simulink model "transmissionlineprotection1"  (R2017a)
settings: Solver=VariableStepAuto  StartTime=0.0  StopTime=0.25  RelTol=1e-3
libraries: powerlib x10, sdolib x6, simulink_extras x3, powerlib_meascontrol x1
settings Model: Creator=abhishek tiwari  LastModifiedBy=abhishek tiwari
settings DataIOCC: ReturnWorkspaceOutputs=on
settings DebuggingCC: UnconnectedInputMsg=none  UnconnectedOutputMsg=none  UnconnectedLineMsg=none
settings ModelReferenceCC: EnableRefExpFcnMdlSchedulingChecks=off
settings SFSimCC: SimUseLocalCustomCode=on
settings RTWCC: RTWUseLocalCustomCode=on

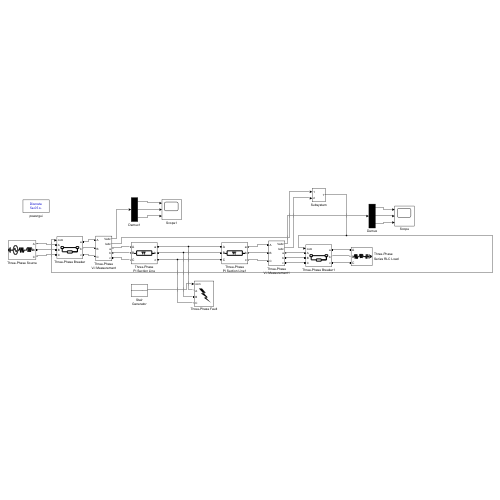
[thumbnail: Simulink's stored preview of the top-level diagram]
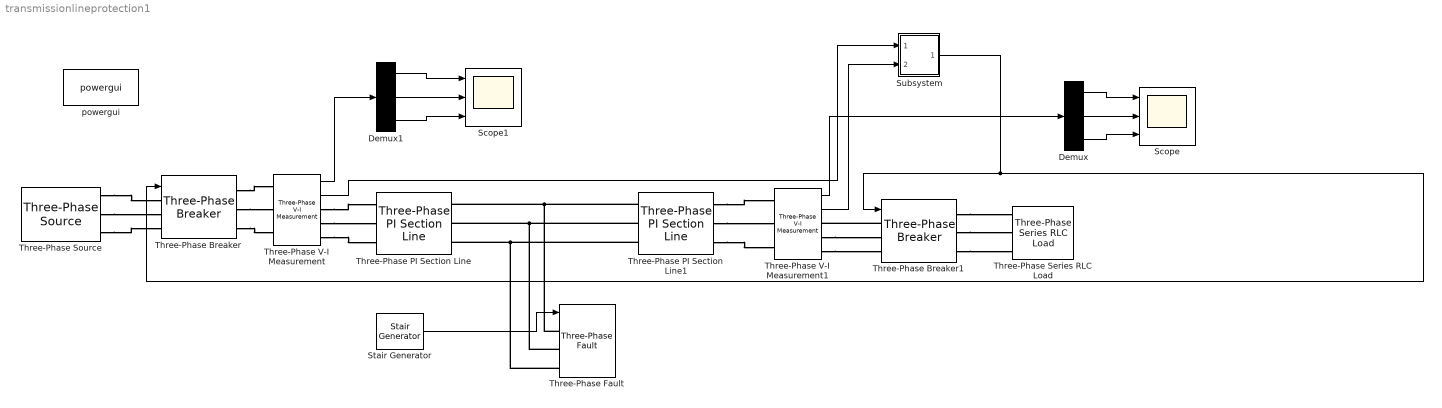
== system transmissionlineprotection1 ==
  Demux : Demux  Outputs=3
  Demux1 : Demux  Outputs=3
  Scope : Scope  NumInputPorts=3
  Scope1 : Scope  NumInputPorts=3
  Stair Generator : powerlib_meascontrol/Pulse & Signal Generators/Stair Generator  t=[0,0.02,0.14,0.2]  e=[0,0,0,0]  Ts=0
  Subsystem : Subsystem
  Three-Phase PI Section Line : powerlib/Elements/Three-Phase PI Section Line  LConnTagsString=a|b|c  RConnTagsString=A|B|C  Length=100  Frequency=50  Resistances=[ 0.01273 0.3864]  Inductances="[ 0.9337e-3  4.1264e-3]"  Capacitances=[12.74e-9 7.751e-9]
  Three-Phase PI Section Line1 : powerlib/Elements/Three-Phase PI Section Line  LConnTagsString=a|b|c  RConnTagsString=A|B|C  Length=100  Frequency=50  Resistances=[ 0.01273 0.3864]  Inductances="[ 0.9337e-3  4.1264e-3]"  Capacitances=[12.74e-9 7.751e-9]
  Three-Phase Series RLC Load : powerlib/Elements/Three-Phase Series RLC Load  LConnTagsString=A|B|C  Configuration=Y (grounded)  NominalVoltage=1000  Vabc=[1e3 1e3 1e3]  Vabcp=[1e3 1e3 1e3]  NominalFrequency=50  UnbalancedPower=off  ActivePower=10e3  InductivePower=100  CapacitivePower=100  Pabc=[10e3 9e3 11e3]  QLabc=[100 90 110]  QCabc=[100 90 110]  Pabcp=[10e3 9e3 11e3]  QLabcp=[100 90 110]  QCabcp=[100 90 110]  Measurements=None  LoadType=constant Z
  Three-Phase V-I Measurement : powerlib/Measurements/Three-Phase V-I Measurement  VoltageMeasurement=phase-to-ground  SetLabelV=off  LabelV=Vabc  Vpu=off  VpuLL=off  CurrentMeasurement=yes  SetLabelI=off  LabelI=Iabc  Ipu=off  Pbase=100e6  Vbase=500e3  OutputType=Complex  PhasorSimulation=off  PSBequivalent=0
  Three-Phase V-I Measurement1 : powerlib/Measurements/Three-Phase V-I Measurement  VoltageMeasurement=phase-to-ground  SetLabelV=off  LabelV=Vabc  Vpu=off  VpuLL=off  CurrentMeasurement=yes  SetLabelI=off  LabelI=Iabc  Ipu=off  Pbase=100e6  Vbase=500e3  OutputType=Complex  PhasorSimulation=off  PSBequivalent=0
  Three-Phase Breaker : powerlib/Elements/Three-Phase Breaker  InitialState=closed  SwitchA=on  SwitchB=on  SwitchC=on  SwitchTimes="[1/60  5/60]"  External=on  BreakerResistance=0.01  SnubberResistance=1e6  SnubberCapacitance=inf  Measurements=None
  Three-Phase Breaker1 : powerlib/Elements/Three-Phase Breaker  InitialState=closed  SwitchA=on  SwitchB=on  SwitchC=on  SwitchTimes="[1/60  5/60]"  External=on  BreakerResistance=0.01  SnubberResistance=1e6  SnubberCapacitance=inf  Measurements=None
  Three-Phase Fault : powerlib/Elements/Three-Phase Fault  InitialStates=0  FaultA=on  FaultB=on  FaultC=on  GroundFault=on  SwitchTimes="[1/60  5/60]"  External=on  SwitchStatus=NaN  FaultResistance=0.001  GroundResistance=0.01  SnubberResistance=1e6  SnubberCapacitance=inf  Measurements=None
  Three-Phase Source : powerlib/Electrical Sources/Three-Phase Source  InternalConnection=Yg  VoltagePhases=off  Voltage=25e3  PhaseAngle=0  Voltage_phases=[25e3 25e3 25e3]/sqrt(3)  PhaseAngles_phases=[0 -120 +120]  Frequency=50  NonIdealSource=on  SpecifyImpedance=on  Resistance=0.8929  Inductance=16.58e-3  ShortCircuitLevel=100e6  BaseVoltage=25e3  XRratio=7  BusType=swing  Pref=10e3  Qref=0  Prefabc=[10e3, 10e3, 10e3]  Qrefabc=[0, 0, 0]  Qmin=-inf  Qmax=inf
  powergui : powerlib/powergui  Priority=1  SimulationMode=Discrete  SampleTime=50e-6  frequency=60  Iterations=50  frequencyindice=50  Pbase=100e6  ErrMax=1e-4  UnitsV=kV  UnitsW=MW  buscounter=0  FunctionMessages=off  echomessages=off  EnableUseOfTLC=off  CurrentSourceSwitches=off  DisableSnubberDevices=off  DisableRonSwitches=off  DisableVfSwitches=off  DisplayEquations=off  AutomaticDiscreteSolvers=off  SolverType=Tustin/Backward Euler (TBE)  Interpol=off  ExternalGateDelay=off  methode=off  Ts=100  x0status=blocks  SPID=on  SwTol=0  HookPort=off  NonlinearTolerance=1e-4  nMaxIteration=100  ContinueOnMaxIteration=off  RestoreLinks=warning  ResistiveCurrentMeasurement=off  Frange=[0:2:500]  Ylog=off  Xlog=on  ShowGrid=off  save=off  variable=ZData  structure=0  ZoomFFT=off  StartTime=0.0  cycles=1  DisplayStyle=1  fundamental=60  FreqAxis=off  MaxFrequency=1000  frequencyindicesteady=1  RmsSteady=1  display=off
  wires:
  Stair Generator/1 -> Three-Phase Fault/1
  Subsystem/1(Out1) -> Three-Phase Breaker1/1, Three-Phase Breaker/1
  Three-Phase V-I Measurement/2 -> Subsystem/1(In1)
  Three-Phase V-I Measurement1/2 -> Subsystem/2(In2)
  Demux/1 -> Scope/1
  Demux/2 -> Scope/2
  Demux/3 -> Scope/3
  Three-Phase V-I Measurement1/1 -> Demux/1
  Demux1/3 -> Scope1/3
  Demux1/1 -> Scope1/1
  Demux1/2 -> Scope1/2
  Three-Phase V-I Measurement/1 -> Demux1/1
  connections:
  Three-Phase Source/RConn1 -- Three-Phase Breaker/LConn1
  Three-Phase Source/RConn2 -- Three-Phase Breaker/LConn2
  Three-Phase Source/RConn3 -- Three-Phase Breaker/LConn3
  Three-Phase Breaker/RConn1 -- Three-Phase V-I Measurement/LConn1
  Three-Phase Breaker/RConn2 -- Three-Phase V-I Measurement/LConn2
  Three-Phase Breaker/RConn3 -- Three-Phase V-I Measurement/LConn3
  Three-Phase V-I Measurement/RConn1 -- Three-Phase PI Section Line/LConn1
  Three-Phase V-I Measurement/RConn2 -- Three-Phase PI Section Line/LConn2
  Three-Phase V-I Measurement/RConn3 -- Three-Phase PI Section Line/LConn3
  Three-Phase PI Section Line1/LConn1 -- Three-Phase Fault/LConn1 -- Three-Phase PI Section Line/RConn1
  Three-Phase PI Section Line1/LConn2 -- Three-Phase Fault/LConn2 -- Three-Phase PI Section Line/RConn2
  Three-Phase PI Section Line1/LConn3 -- Three-Phase Fault/LConn3 -- Three-Phase PI Section Line/RConn3
  Three-Phase PI Section Line1/RConn1 -- Three-Phase V-I Measurement1/LConn1
  Three-Phase PI Section Line1/RConn2 -- Three-Phase V-I Measurement1/LConn2
  Three-Phase PI Section Line1/RConn3 -- Three-Phase V-I Measurement1/LConn3
  Three-Phase Breaker1/LConn1 -- Three-Phase V-I Measurement1/RConn1
  Three-Phase V-I Measurement1/RConn2 -- Three-Phase Breaker1/LConn2
  Three-Phase V-I Measurement1/RConn3 -- Three-Phase Breaker1/LConn3
  Three-Phase Breaker1/RConn1 -- Three-Phase Series RLC Load/LConn1
  Three-Phase Breaker1/RConn2 -- Three-Phase Series RLC Load/LConn2
  Three-Phase Breaker1/RConn3 -- Three-Phase Series RLC Load/LConn3

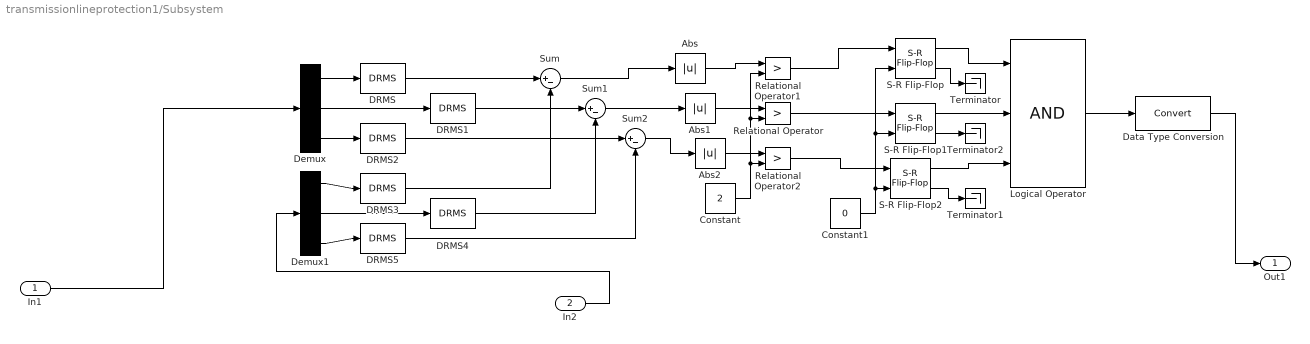
== system transmissionlineprotection1/Subsystem ==
  In1 : Inport
  In2 : Inport  Port=2
  Abs : Abs
  Abs1 : Abs
  Abs2 : Abs
  Constant : Constant  Value=2
  Constant1 : Constant  Value=0  OutDataTypeStr=boolean
  DRMS{,1..5} (6 alike) : sdolib/RMS Blocks/DRMS  Ts=1
  Data Type Conversion : DataTypeConversion
  Demux : Demux  Outputs=3
  Demux1 : Demux  Outputs=3
  Logical Operator : Logic  Inputs=3  AllPortsSameDT=off  OutDataTypeStr=boolean
  Relational Operator : RelationalOperator  Operator=>  OutDataTypeStr=boolean  RndMeth=Simplest
  Relational Operator1 : RelationalOperator  Operator=>  OutDataTypeStr=boolean  RndMeth=Simplest
  Relational Operator2 : RelationalOperator  Operator=>  OutDataTypeStr=boolean  RndMeth=Simplest
  S-R Flip-Flop : simulink_extras/Flip Flops/S-R Flip-Flop  initial_condition=0
  S-R Flip-Flop1 : simulink_extras/Flip Flops/S-R Flip-Flop  initial_condition=0
  S-R Flip-Flop2 : simulink_extras/Flip Flops/S-R Flip-Flop  initial_condition=0
  Sum : Sum  Inputs=|+-
  Sum1 : Sum  Inputs=|+-
  Sum2 : Sum  Inputs=|+-
  Terminator : Terminator
  Terminator1 : Terminator
  Terminator2 : Terminator
  Out1 : Outport
  wires:
  S-R Flip-Flop/2 -> Terminator/1
  Logical Operator/1 -> Data Type Conversion/1
  Abs/1 -> Relational Operator1/1
  DRMS1/1 -> Sum1/1
  Abs2/1 -> Relational Operator2/1
  In1/1 -> Demux/1
  Sum2/1 -> Abs2/1
  In2/1 -> Demux1/1
  Demux1/3 -> DRMS5/1
  Constant1/1 -> S-R Flip-Flop/2, S-R Flip-Flop1/2, S-R Flip-Flop2/2
  S-R Flip-Flop1/1 -> Logical Operator/2
  Data Type Conversion/1 -> Out1/1
  Sum1/1 -> Abs1/1
  Demux1/1 -> DRMS3/1
  DRMS/1 -> Sum/1
  Abs1/1 -> Relational Operator/1
  Demux/2 -> DRMS1/1
  DRMS3/1 -> Sum/2
  S-R Flip-Flop2/1 -> Logical Operator/3
  Relational Operator2/1 -> S-R Flip-Flop2/1
  Constant/1 -> Relational Operator1/2, Relational Operator/2, Relational Operator2/2
  DRMS5/1 -> Sum2/2
  Relational Operator1/1 -> S-R Flip-Flop/1
  Relational Operator/1 -> S-R Flip-Flop1/1
  Demux/1 -> DRMS/1
  DRMS2/1 -> Sum2/1
  S-R Flip-Flop1/2 -> Terminator2/1
  S-R Flip-Flop2/2 -> Terminator1/1
  Demux/3 -> DRMS2/1
  DRMS4/1 -> Sum1/2
  S-R Flip-Flop/1 -> Logical Operator/1
  Sum/1 -> Abs/1
  Demux1/2 -> DRMS4/1
